simulink model "lookupnd_out_table_test"  (Simulink 8.4)
settings: Solver=ode45  StartTime=0.0  StopTime=10.0  RelTol=1e-3
settings Model: Creator=arnaud  LastModifiedBy=arnaud
settings DataIOCC: SaveFormat=Structure

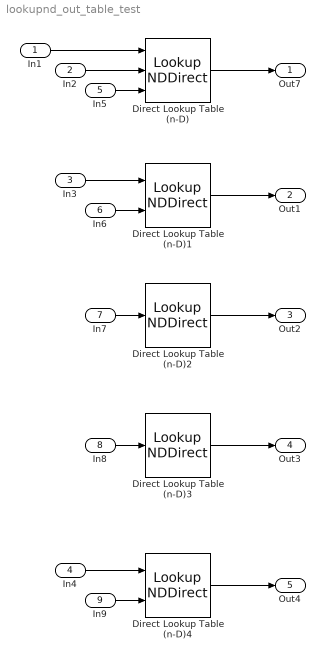
== system lookupnd_out_table_test ==
  In1 : Inport  PortDimensions=1
  In2 : Inport  Port=2  PortDimensions=1
  In3 : Inport  Port=3  PortDimensions=1
  In4 : Inport  Port=4  PortDimensions=1
  In5 : Inport  Port=5  PortDimensions=[2 3]
  In6 : Inport  Port=6  PortDimensions=4
  In7 : Inport  Port=7  PortDimensions=5
  In8 : Inport  Port=8  PortDimensions=[2 3]
  In9 : Inport  Port=9  PortDimensions=[ 4 5]
  Direct Lookup Table (n-D) : LookupNDDirect  TableIsInput=on
  Direct Lookup Table (n-D)1 : LookupNDDirect  NumberOfTableDimensions=1  TableIsInput=on  Table=[4 5 6]
  Direct Lookup Table (n-D)2 : LookupNDDirect  NumberOfTableDimensions=1  InputsSelectThisObjectFromTable=Column  TableIsInput=on  Table=[4 5 6]
  Direct Lookup Table (n-D)3 : LookupNDDirect  InputsSelectThisObjectFromTable=2-D Matrix  TableIsInput=on  Table=[4 5 6; 7 8 9]
  Direct Lookup Table (n-D)4 : LookupNDDirect  InputsSelectThisObjectFromTable=Column  TableIsInput=on  Table=[4 5 6; 7 8 9]
  Out7 : Outport
  Out1 : Outport  Port=2
  Out2 : Outport  Port=3
  Out3 : Outport  Port=4
  Out4 : Outport  Port=5
  wires:
  In1/1 -> Direct Lookup Table (n-D)/1
  In2/1 -> Direct Lookup Table (n-D)/2
  Direct Lookup Table (n-D)/1 -> Out7/1
  In3/1 -> Direct Lookup Table (n-D)1/1
  Direct Lookup Table (n-D)1/1 -> Out1/1
  Direct Lookup Table (n-D)2/1 -> Out2/1
  Direct Lookup Table (n-D)3/1 -> Out3/1
  Direct Lookup Table (n-D)4/1 -> Out4/1
  In4/1 -> Direct Lookup Table (n-D)4/1
  In5/1 -> Direct Lookup Table (n-D)/3
  In6/1 -> Direct Lookup Table (n-D)1/2
  In7/1 -> Direct Lookup Table (n-D)2/1
  In8/1 -> Direct Lookup Table (n-D)3/1
  In9/1 -> Direct Lookup Table (n-D)4/2
